simulink model "M2C_IM_CL_V1_NCADMM_Sim"  (R2023a)
settings: Solver=ode4  StartTime=0.0  StopTime=t_sim  FixedStep=tsim  RelTol=1e-3
model workspace (MAT data in the model file):
  global_can_baud_rate = '1000000'
  global_ip_addresses : object (value not decoded)
values from neighbouring files (symbols this model uses):
  A = [1 1 1 0 0 0 ... (first row only)    [M2C_init.m]    (also in MMCC_Sim_Script_BCD_activeset.m = -[1 0 0 1 0 0 1 0 0; 0 1 0 0 1 0 0 1 0; 0 0 1 0 0 1 0 0 1; -; MMCC_Sim_Script_BCD_activeset_LH.m = -[1 0 0 1 0 0 1 0 0; 0 1 0 0 1 0 0 1 0; 0 0 1 0 0 1 0 0 1; -)
  A11 = -(1/tau_sig)*eye(2)    [M2C_init.m]
  A21 = (Lm/tau_r)*eye(2)    [M2C_init.m]
  A_admm = zeros(2*Np, Np)    [M2C_init.m]
  A_cc = [1 0 ... (first row only)    [M2C_init.m]
  b_admm_1 = imax_admm*ones(2*Np,1)    [M2C_init.m]
  b_cc = Vmax_cc*ones(4,1)    [M2C_init.m]
  c_admm = -imax_admm*ones(Np,1)    [M2C_init.m]
  C_obs = [eye(2) zeros(2)]    [M2C_init.m]
  C_sm = 987e-6    (= 0.000987)    [M2C_init.m]
  G_cc = [1 1 ... (first row only)    [M2C_init.m]
  J_imag = [0 -1 ... (first row only)    [M2C_init.m]
  K_obsm = K_obs2'    [M2C_init.m]
  K_obsp = K_obs1'    [M2C_init.m]
  kr = Lm/Lr    (= 0.989061842659)    [M2C_init.m]
  L = 5e-3    (= 0.005)    [M2C_init.m]    (also in MMCC_Sim_Script_BCD_activeset.m = 0.02; MMCC_Sim_Script_BCD_activeset_LH.m = 0.02)
  Lsigmar = 2.6e-3    (= 0.0026)    [M2C_init.m]
  Lsigmas = 2.6e-3    (= 0.0026)    [M2C_init.m]
  N = [1/sqrt(3) 0;-1/(2*sqrt(3)) 1/2;-1/(2*sqrt(3)) -1/2;-1/sqrt(3) 0;1/(2*sqrt(3)) -1/2;1/(2*sqrt(3)) 1/2]    [M2C_init.m]    (also in MMCC_Sim_Script_BCD_activeset.m = null(A,'rational'); MMCC_Sim_Script_BCD_activeset_LH.m = [-0.4430   -0.4780    0.0994    0.0994)
  n = 4    [M2C_init.m]
  p = 2    [M2C_init.m]
  phirN = 1*Vb/ws_nom    [M2C_init.m]
  prmt_ADMM = [n, lambda_z, rho, lambda_e, C_sm, Np, imax_admm]    [M2C_init.m]
  prmt_bkpsi = [ts, Np, lambda_o, imax_admm]    [M2C_init.m]
  prmt_CCMPC = [ts, L, lambda_u, lambda_i, R, e]    [M2C_init.m]
  prmt_OBS = [ts, kr, sigma, Ls, tau_r]    [M2C_init.m]
  R = 0.2    [M2C_init.m]    (also in MMCC_Sim_Script_BCD_activeset.m = 0.001; MMCC_Sim_Script_BCD_activeset_LH.m = 0.001)
  Rr = 1.8    [M2C_init.m]
  Rs = 1.8    [M2C_init.m]
  Rsig = Rs + Rr*kr^2    (= 3.56083799149)    [M2C_init.m]
  SN = PN/FPn    (= 3703.7037037)    [M2C_init.m]
  T = [An ... (first row only)    [M2C_init.m]    (also in MMCC_Sim_Script_BCD_activeset.m = [1   0 ; -1/2  sqrt(3)/2; -1/2  -sqrt(3)/2]; MMCC_Sim_Script_BCD_activeset_LH.m = [1   0 ; -1/2  sqrt(3)/2; -1/2  -sqrt(3)/2])
  t_arranque = t_flux + 5/(dam*wn_flux) + 0.4    [M2C_init.m]
  t_flux = t_maq + 0.1    (= 0.3)    [M2C_init.m]
  t_load = t_arranque    [M2C_init.m]
  Tab0 = (1/3)*[2 -1 -1 ... (first row only)    [M2C_init.m]
  Tabc = [1 0; -.5 sqrt(3)/2; -.5 -sqrt(3)/2]    [M2C_init.m]
  tau_r = Lr/Rr    (= 0.132055555556)    [M2C_init.m]
  TN = PN/(nN*pi/30)    (= 19.7571653493)    [M2C_init.m]
  ts = 1/fs    (= 0.000166666666667)    [M2C_init.m]
  tsim = ts/40    (= 4.16666666667e-06)    [M2C_init.m]
  Vc0 = n*Vc_sm    (= 520)    [M2C_init.m]    (also in MMCC_Sim_Script_BCD_activeset.m = 18000; MMCC_Sim_Script_BCD_activeset_LH.m = 18000)
  Vc_sm = 130    [M2C_init.m]
  Vdc = n*Vc_sm    (= 520)    [M2C_init.m]
undefined symbols (not defined in the file or in its folder): Down, M2C_ADMM_Init_IM_V1, plecs, Up
libraries: spsIGBTDiodeLib x48, spsVoltageMeasurementLib x36, spsSeriesRLCBranchLib x30, spsCurrentMeasurementLib x10, eePwmGenerator x6, rtlab x3, dspstat3 x2, spsControlledVoltageSourceLib x2, spsDCVoltageSourceLib x2, opal_lib x1, dspfdesign x1, spsMeanLib x1
(part 3 of 6)

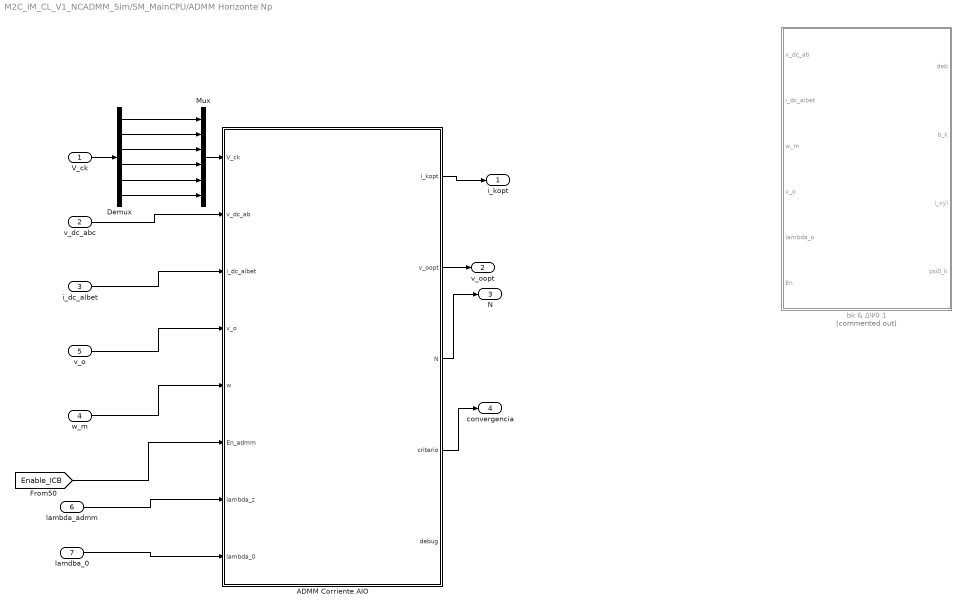
== system M2C_IM_CL_V1_NCADMM_Sim/SM_MainCPU/ADMM Horizonte Np ==
  V_ck : Inport
  v_dc_abc : Inport  Port=2
  i_dc_albet : Inport  Port=3
  w_m : Inport  Port=4
  v_o : Inport  Port=5
  lambda_admm : Inport  Port=6
  lamdba_0 : Inport  Port=7
  ADMM Corriente AIO : MATLAB Function  TreatAsAtomicUnit=on  SystemSampleTime=ts
  Demux : Demux  Outputs=6
  Mux : Mux  Inputs=6
  bk & ΔΨ0 1 : MATLAB Function  Commented=on  TreatAsAtomicUnit=on  SystemSampleTime=ts
  i_kopt : Outport
  v_oopt : Outport  Port=2
  N : Outport  Port=3
  convergencia : Outport  Port=4
  wires:
  V_ck/1 -> Demux/1
  Demux/1 -> Mux/1
  Demux/2 -> Mux/2
  Demux/3 -> Mux/3
  Demux/4 -> Mux/4
  Demux/5 -> Mux/5
  Demux/6 -> Mux/6
  v_o/1 -> ADMM Corriente AIO/4(v_o)
  i_dc_albet/1 -> ADMM Corriente AIO/3(i_dc_albet)
  v_dc_abc/1 -> ADMM Corriente AIO/2(v_dc_ab)
  ADMM Corriente AIO/1(i_kopt) -> i_kopt/1
  ADMM Corriente AIO/3(N) -> N/1
  ADMM Corriente AIO/4(criterio) -> convergencia/1
  [Enable_ICB] -> ADMM Corriente AIO/6(En_admm)
  w_m/1 -> ADMM Corriente AIO/5(w)
  Mux/1 -> ADMM Corriente AIO/1(V_ck)
  lambda_admm/1 -> ADMM Corriente AIO/7(lambda_z)
  lamdba_0/1 -> ADMM Corriente AIO/8(lambda_0)
  ADMM Corriente AIO/2(v_oopt) -> v_oopt/1

== system M2C_IM_CL_V1_NCADMM_Sim/SM_MainCPU/Corrientes ==
  1 : Inport
  2 : Inport  Port=2
  3 : Inport  Port=3
  4 : Inport  Port=4
  " 1 " : DataTypeConversion
  " 2 " : DataTypeConversion
  " 3 " : DataTypeConversion
  " 4 " : DataTypeConversion
  " InputMux " : Mux
  " S-Function " : S-Function  FunctionName=plecs  SFunctionDeploymentMode=off  EnableBusSupport=off
  wires:
  " InputMux "/1 -> " S-Function "/1
  1/1 -> " 1 "/1
  " 1 "/1 -> " InputMux "/1
  2/1 -> " 2 "/1
  " 2 "/1 -> " InputMux "/2
  3/1 -> " 3 "/1
  " 3 "/1 -> " InputMux "/3
  4/1 -> " 4 "/1
  " 4 "/1 -> " InputMux "/4

== system M2C_IM_CL_V1_NCADMM_Sim/SM_MainCPU/Entrada ==
  1 : Inport
  2 : Inport  Port=2
  " 1 " : DataTypeConversion
  " 2 " : DataTypeConversion
  " InputMux " : Mux  Inputs=2
  " S-Function " : S-Function  FunctionName=plecs  SFunctionDeploymentMode=off  EnableBusSupport=off
  wires:
  " InputMux "/1 -> " S-Function "/1
  1/1 -> " 1 "/1
  " 1 "/1 -> " InputMux "/1
  2/1 -> " 2 "/1
  " 2 "/1 -> " InputMux "/2

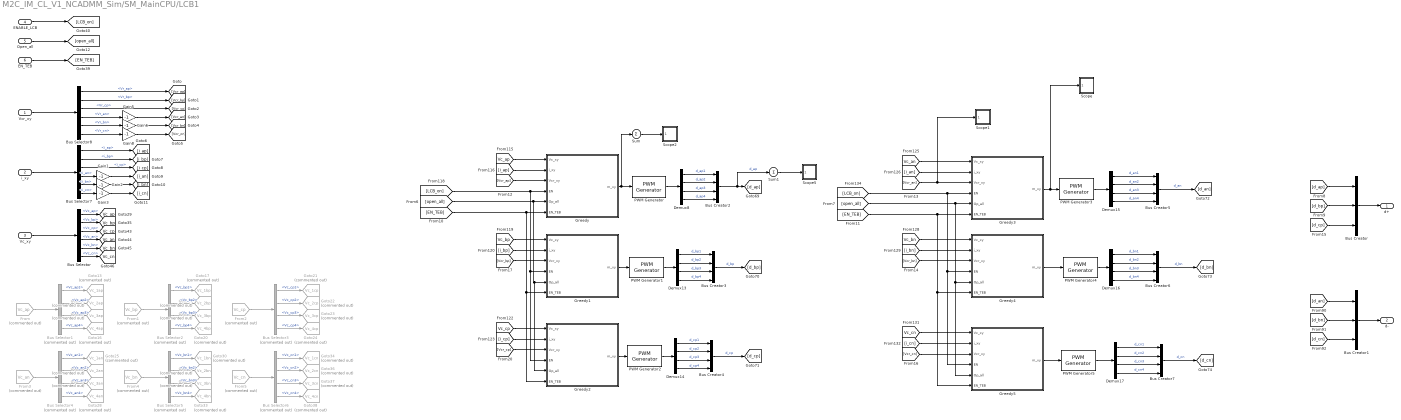
== system M2C_IM_CL_V1_NCADMM_Sim/SM_MainCPU/LCB1 ==
  Vcr_xy : Inport
  i_xy : Inport  Port=2
  Vc_xy : Inport  Port=3
  ENABLE_LCB : Inport  Port=4
  Open_all : Inport  Port=5
  EN_TEB : Inport  Port=6
  Bus Creator : BusCreator  Inputs=3
  Bus Creator1 : BusCreator  Inputs=3
  Bus Creator{2..7} (6 alike) : BusCreator  Inputs=4
  Bus Selector : BusSelector  OutputSignals=Vc_ap,Vc_bp,Vc_cp,Vc_an,Vc_bn,Vc_cn
  Bus Selector1 : BusSelector  Commented=on  OutputSignals=Vc_ap1,Vc_ap2,Vc_ap3,Vc_ap4
  Bus Selector2 : BusSelector  Commented=on  OutputSignals=Vc_bp1,Vc_bp2,Vc_bp3,Vc_bp4
  Bus Selector3 : BusSelector  Commented=on  OutputSignals=Vc_cp1,Vc_cp2,Vc_cp3,Vc_cp4
  Bus Selector4 : BusSelector  Commented=on  OutputSignals=Vc_an1,Vc_an2,Vc_an3,Vc_an4
  Bus Selector5 : BusSelector  Commented=on  OutputSignals=Vc_bn1,Vc_bn2,Vc_bn3,Vc_bn4
  Bus Selector6 : BusSelector  Commented=on  OutputSignals=Vc_cn1,Vc_cn2,Vc_cn3,Vc_cn4
  Bus Selector7 : BusSelector  OutputSignals=i_ap,i_bp,i_cp,i_an,i_bn,i_cn
  Bus Selector8 : BusSelector  OutputSignals=Vr_ap,Vr_bp,Vr_cp,Vr_an,Vr_bn,Vr_cn
  Demux{8,13..17} (6 alike) : Demux
  From : From  Commented=on  GotoTag=Vc_ap  TagVisibility=global
  From1 : From  Commented=on  GotoTag=Vc_bp  TagVisibility=global
  From2 : From  Commented=on  GotoTag=Vc_cp  TagVisibility=global
  From3 : From  Commented=on  GotoTag=Vc_an  TagVisibility=global
  From4 : From  Commented=on  GotoTag=Vc_bn  TagVisibility=global
  From5 : From  Commented=on  GotoTag=Vc_cn  TagVisibility=global
  Gain{1..3,5..6,8} (6 alike) : Gain  Gain=-1
  Goto13 : Goto  Commented=on  GotoTag=Vc_1ap  TagVisibility=global
  Goto14 : Goto  Commented=on  GotoTag=Vc_2ap  TagVisibility=global
  Goto15 : Goto  Commented=on  GotoTag=Vc_3ap  TagVisibility=global
  Goto16 : Goto  Commented=on  GotoTag=Vc_4ap  TagVisibility=global
  Goto17 : Goto  Commented=on  GotoTag=Vc_1bp  TagVisibility=global
  Goto18 : Goto  Commented=on  GotoTag=Vc_2bp  TagVisibility=global
  Goto19 : Goto  Commented=on  GotoTag=Vc_3bp  TagVisibility=global
  Goto20 : Goto  Commented=on  GotoTag=Vc_4bp  TagVisibility=global
  Goto21 : Goto  Commented=on  GotoTag=Vc_1cp  TagVisibility=global
  Goto22 : Goto  Commented=on  GotoTag=Vc_2cp  TagVisibility=global
  Goto23 : Goto  Commented=on  GotoTag=Vc_3cp  TagVisibility=global
  Goto24 : Goto  Commented=on  GotoTag=Vc_4cp  TagVisibility=global
  Goto25 : Goto  Commented=on  GotoTag=Vc_1an  TagVisibility=global
  Goto26 : Goto  Commented=on  GotoTag=Vc_2an  TagVisibility=global
  Goto27 : Goto  Commented=on  GotoTag=Vc_3an  TagVisibility=global
  Goto28 : Goto  Commented=on  GotoTag=Vc_4an  TagVisibility=global
  Goto30 : Goto  Commented=on  GotoTag=Vc_1bn  TagVisibility=global
  Goto31 : Goto  Commented=on  GotoTag=Vc_2bn  TagVisibility=global
  Goto32 : Goto  Commented=on  GotoTag=Vc_3bn  TagVisibility=global
  Goto33 : Goto  Commented=on  GotoTag=Vc_4bn  TagVisibility=global
  Goto34 : Goto  Commented=on  GotoTag=Vc_1cn  TagVisibility=global
  Goto36 : Goto  Commented=on  GotoTag=Vc_2cn  TagVisibility=global
  Goto37 : Goto  Commented=on  GotoTag=Vc_3cn  TagVisibility=global
  Goto38 : Goto  Commented=on  GotoTag=Vc_4cn  TagVisibility=global
  Greedy : MATLAB Function  TreatAsAtomicUnit=on
  Greedy1 : MATLAB Function  TreatAsAtomicUnit=on
  Greedy2 : MATLAB Function  TreatAsAtomicUnit=on
  Greedy3 : MATLAB Function  TreatAsAtomicUnit=on
  Greedy4 : MATLAB Function  TreatAsAtomicUnit=on
  Greedy5 : MATLAB Function  TreatAsAtomicUnit=on
  PWM Generator{,1..5} (6 alike) : eePwmGenerator/PWM Generator  CarrCount=Up-Down  Tper=ts*0.5  Tdelay=0  Ts=tsim
  Scope : Subsystem  LoadFcn=plecs('sl', 300);  InitFcn=plecs('sl', 314);  StartFcn=plecs('sl', 308);  StopFcn=plecs('sl', 309);  mask{Settings=<binary blob, 1052 chars, not shown>}
      mask init:
      | plecs('sl', 315);
      settings: CopyFcn=plecs('sl', 303);  DeleteFcn=plecs('sl', 305);  UndoDeleteFcn=plecs('sl', 306);  PreSaveFcn=plecs('sl', 311);  NameChangeFcn=plecs('sl', 310);  DestroyFcn=plecs('sl', 307);  OpenFcn=plecs('sl', 302);  ErrorFcn=plerrorfcn
      mask Display: plot([0.1 0.9 0.9 0.1 0.1], [0.9 0.9 0.5 0.5 0.9])
  Scope1 : Subsystem  LoadFcn=plecs('sl', 300);  InitFcn=plecs('sl', 314);  StartFcn=plecs('sl', 308);  StopFcn=plecs('sl', 309);  mask{Settings=<binary blob, 1052 chars, not shown>}
      mask init:
      | plecs('sl', 315);
      settings: CopyFcn=plecs('sl', 303);  DeleteFcn=plecs('sl', 305);  UndoDeleteFcn=plecs('sl', 306);  PreSaveFcn=plecs('sl', 311);  NameChangeFcn=plecs('sl', 310);  DestroyFcn=plecs('sl', 307);  OpenFcn=plecs('sl', 302);  ErrorFcn=plerrorfcn
      mask Display: plot([0.1 0.9 0.9 0.1 0.1], [0.9 0.9 0.5 0.5 0.9])
  Scope2 : Subsystem  LoadFcn=plecs('sl', 300);  InitFcn=plecs('sl', 314);  StartFcn=plecs('sl', 308);  StopFcn=plecs('sl', 309);  mask{Settings=<binary blob, 1020 chars, not shown>}
      mask init:
      | plecs('sl', 315);
      settings: CopyFcn=plecs('sl', 303);  DeleteFcn=plecs('sl', 305);  UndoDeleteFcn=plecs('sl', 306);  PreSaveFcn=plecs('sl', 311);  NameChangeFcn=plecs('sl', 310);  DestroyFcn=plecs('sl', 307);  OpenFcn=plecs('sl', 302);  ErrorFcn=plerrorfcn
      mask Display: plot([0.1 0.9 0.9 0.1 0.1], [0.9 0.9 0.5 0.5 0.9])
  Scope5 : Subsystem  LoadFcn=plecs('sl', 300);  InitFcn=plecs('sl', 314);  StartFcn=plecs('sl', 308);  StopFcn=plecs('sl', 309);  mask{Settings=<binary blob, 1020 chars, not shown>}
      mask init:
      | plecs('sl', 315);
      settings: CopyFcn=plecs('sl', 303);  DeleteFcn=plecs('sl', 305);  UndoDeleteFcn=plecs('sl', 306);  PreSaveFcn=plecs('sl', 311);  NameChangeFcn=plecs('sl', 310);  DestroyFcn=plecs('sl', 307);  OpenFcn=plecs('sl', 302);  ErrorFcn=plerrorfcn
      mask Display: plot([0.1 0.9 0.9 0.1 0.1], [0.9 0.9 0.5 0.5 0.9])
  Sum : Sum  Inputs=+
  Sum1 : Sum  Inputs=+
  d+ : Outport
  d- : Outport  Port=2
  tag scope: Vc_an=global, Vc_ap=global, Vc_bn=global, Vc_bp=global, Vc_cn=global, Vc_cp=global
  wires:
  Bus Creator1/1 -> d-/1
  Bus Selector8/5 -> Gain6/1  "<Vr_bn>"
  Bus Selector8/6 -> Gain8/1  "<Vr_cn>"
  Bus Selector8/4 -> Gain5/1  "<Vr_an>"
  Bus Creator/1 -> d+/1
  Gain3/1 -> [i_cn]
  Gain2/1 -> [i_bn]
  Gain1/1 -> [i_an]
  Bus Selector7/3 -> [i_cp]  "<i_cp>"
  Bus Selector7/2 -> [i_bp]  "<i_bp>"
  Bus Selector7/1 -> [i_ap]  "<i_ap>"
  Bus Selector7/4 -> Gain1/1  "<i_an>"
  Bus Selector7/6 -> Gain3/1  "<i_cn>"
  Bus Selector7/5 -> Gain2/1  "<i_bn>"
  Bus Selector/3 -> [Vc_cp]  "<Vc_cp>"
  Bus Selector/2 -> [Vc_bp]  "<Vc_bp>"
  Bus Selector/6 -> [Vc_cn]  "<Vc_cn>"
  Bus Selector/4 -> [Vc_an]  "<Vc_an>"
  Bus Selector/5 -> [Vc_bn]  "<Vc_bn>"
  Bus Selector/1 -> [Vc_ap]  "<Vc_ap>"
  Bus Selector1/1 -> Goto13/1  "<Vc_ap1>"
  Bus Selector1/2 -> Goto14/1  "<Vc_ap2>"
  Bus Selector1/3 -> Goto15/1  "<Vc_ap3>"
  Bus Selector1/4 -> Goto16/1  "<Vc_ap4>"
  Bus Selector2/4 -> Goto20/1  "<Vc_bp4>"
  Bus Selector2/2 -> Goto18/1  "<Vc_bp2>"
  Bus Selector2/1 -> Goto17/1  "<Vc_bp1>"
  Bus Selector2/3 -> Goto19/1  "<Vc_bp3>"
  Bus Selector3/4 -> Goto24/1  "<Vc_cp4>"
  Bus Selector3/2 -> Goto22/1  "<Vc_cp2>"
  Bus Selector3/1 -> Goto21/1  "<Vc_cp1>"
  Bus Selector3/3 -> Goto23/1  "<Vc_cp3>"
  Bus Selector4/4 -> Goto28/1  "<Vc_an4>"
  Bus Selector4/2 -> Goto26/1  "<Vc_an2>"
  Bus Selector4/1 -> Goto25/1  "<Vc_an1>"
  Bus Selector4/3 -> Goto27/1  "<Vc_an3>"
  Bus Selector5/4 -> Goto33/1  "<Vc_bn4>"
  Bus Selector5/2 -> Goto31/1  "<Vc_bn2>"
  Bus Selector5/1 -> Goto30/1  "<Vc_bn1>"
  Bus Selector5/3 -> Goto32/1  "<Vc_bn3>"
  Bus Selector6/4 -> Goto38/1  "<Vc_cn4>"
  Bus Selector6/2 -> Goto36/1  "<Vc_cn2>"
  Bus Selector6/1 -> Goto34/1  "<Vc_cn1>"
  Bus Selector6/3 -> Goto37/1  "<Vc_cn3>"
  [d_ap] -> Bus Creator/1
  [d_bp] -> Bus Creator/2
  [d_cp] -> Bus Creator/3
  [d_an] -> Bus Creator1/1
  [d_bn] -> Bus Creator1/2
  [d_cn] -> Bus Creator1/3
  [Vc_ap] -> Greedy/1(Vc_xy)
  [i_ap] -> Greedy/2(i_xy)
  Bus Selector8/2 -> [Vcr_bp]  "<Vr_bp>"
  Bus Selector8/3 -> [Vcr_cp]  "<Vr_cp>"
  Gain5/1 -> [Vcr_an]
  Gain6/1 -> [Vcr_bn]
  Gain8/1 -> [Vcr_cn]
  Bus Selector8/1 -> [Vcr_ap]  "<Vr_ap>"
  [Vcr_ap] -> Greedy/3(Vcr_xy)
  Vcr_xy/1 -> Bus Selector8/1
  Demux15/1 -> Bus Creator5/1  "d_an1"
  Demux15/2 -> Bus Creator5/2  "d_an2"
  Demux15/3 -> Bus Creator5/3  "d_an3"
  Demux15/4 -> Bus Creator5/4  "d_an4"
  Bus Creator5/1 -> [d_an]  "d_an"
  Demux8/3 -> Bus Creator2/3  "d_ap3"
  Demux8/1 -> Bus Creator2/1  "d_ap1"
  Demux8/2 -> Bus Creator2/2  "d_ap2"
  Demux8/4 -> Bus Creator2/4  "d_ap4"
  Demux13/4 -> Bus Creator3/4  "d_bp4"
  Demux13/2 -> Bus Creator3/2  "d_bp2"
  Demux13/1 -> Bus Creator3/1  "d_bp1"
  Demux13/3 -> Bus Creator3/3  "d_bp3"
  Demux14/3 -> Bus Creator4/3  "d_cp3"
  Demux14/1 -> Bus Creator4/1  "d_cp1"
  Demux14/2 -> Bus Creator4/2  "d_cp2"
  Demux14/4 -> Bus Creator4/4  "d_cp4"
  Bus Creator4/1 -> [d_cp]  "d_cp"
  Bus Creator3/1 -> [d_bp]  "d_bp"
  Bus Creator2/1 -> Sum1/1, [d_ap]  "d_ap"
  Bus Creator6/1 -> [d_bn]  "d_bn"
  Demux16/4 -> Bus Creator6/4  "d_bn4"
  Demux16/3 -> Bus Creator6/3  "d_bn3"
  Demux16/2 -> Bus Creator6/2  "d_bn2"
  Demux16/1 -> Bus Creator6/1  "d_bn1"
  Demux17/1 -> Bus Creator7/1  "d_cn1"
  Demux17/2 -> Bus Creator7/2  "d_cn2"
  Demux17/3 -> Bus Creator7/3  "d_cn3"
  Demux17/4 -> Bus Creator7/4  "d_cn4"
  Bus Creator7/1 -> [d_cn]  "d_cn"
  Vc_xy/1 -> Bus Selector/1
  From/1 -> Bus Selector1/1
  From1/1 -> Bus Selector2/1
  From2/1 -> Bus Selector3/1
  From3/1 -> Bus Selector4/1
  From4/1 -> Bus Selector5/1
  From5/1 -> Bus Selector6/1
  i_xy/1 -> Bus Selector7/1
  ENABLE_LCB/1 -> [LCB_on]
  Greedy/1(m_xy) -> Sum/1, PWM Generator/1
  Open_all/1 -> [open_all]
  Greedy1/1(m_xy) -> PWM Generator1/1
  Greedy2/1(m_xy) -> PWM Generator2/1
  [LCB_on] -> Greedy/4(EN), Greedy2/4(EN), Greedy1/4(EN)
  [open_all] -> Greedy2/5(Op_all), Greedy1/5(Op_all), Greedy/5(Op_all)
  EN_TEB/1 -> [EN_TEB]
  [EN_TEB] -> Greedy2/6(EN_TEB), Greedy1/6(EN_TEB), Greedy/6(EN_TEB)
  [Vc_bp] -> Greedy1/1(Vc_xy)
  [i_bp] -> Greedy1/2(i_xy)
  [Vcr_bp] -> Greedy1/3(Vcr_xy)
  [Vc_cp] -> Greedy2/1(Vc_xy)
  [i_cp] -> Greedy2/2(i_xy)
  [Vcr_cp] -> Greedy2/3(Vcr_xy)
  Greedy3/1(m_xy) -> Scope/1(1), PWM Generator3/1
  [Vc_an] -> Greedy3/1(Vc_xy)
  [i_an] -> Greedy3/2(i_xy)
  [Vcr_an] -> Scope1/1(1), Greedy3/3(Vcr_xy)
  [EN_TEB] -> Greedy3/6(EN_TEB), Greedy5/6(EN_TEB), Greedy4/6(EN_TEB)
  [LCB_on] -> Greedy3/4(EN), Greedy5/4(EN), Greedy4/4(EN)
  [open_all] -> Greedy3/5(Op_all), Greedy5/5(Op_all), Greedy4/5(Op_all)
  Greedy4/1(m_xy) -> PWM Generator4/1
  [Vc_bn] -> Greedy4/1(Vc_xy)
  [i_bn] -> Greedy4/2(i_xy)
  [Vcr_bn] -> Greedy4/3(Vcr_xy)
  Greedy5/1(m_xy) -> PWM Generator5/1
  [Vc_cn] -> Greedy5/1(Vc_xy)
  [i_cn] -> Greedy5/2(i_xy)
  [Vcr_cn] -> Greedy5/3(Vcr_xy)
  PWM Generator/1 -> Demux8/1
  PWM Generator1/1 -> Demux13/1
  PWM Generator2/1 -> Demux14/1
  PWM Generator3/1 -> Demux15/1
  PWM Generator4/1 -> Demux16/1
  PWM Generator5/1 -> Demux17/1
  Sum/1 -> Scope2/1(1)
  Sum1/1 -> Scope5/1(1)

== system M2C_IM_CL_V1_NCADMM_Sim/SM_MainCPU/Salida ==
  1 : Inport
  2 : Inport  Port=2
  3 : Inport  Port=3
  4 : Inport  Port=4
  5 : Inport  Port=5
  " 1 " : DataTypeConversion
  " 2 " : DataTypeConversion
  " 3 " : DataTypeConversion
  " 4 " : DataTypeConversion
  " 5 " : DataTypeConversion
  " InputMux " : Mux  Inputs=5
  " S-Function " : S-Function  FunctionName=plecs  SFunctionDeploymentMode=off  EnableBusSupport=off
  wires:
  " InputMux "/1 -> " S-Function "/1
  1/1 -> " 1 "/1
  " 1 "/1 -> " InputMux "/1
  2/1 -> " 2 "/1
  " 2 "/1 -> " InputMux "/2
  3/1 -> " 3 "/1
  " 3 "/1 -> " InputMux "/3
  4/1 -> " 4 "/1
  " 4 "/1 -> " InputMux "/4
  5/1 -> " 5 "/1
  " 5 "/1 -> " InputMux "/5

== system M2C_IM_CL_V1_NCADMM_Sim/SM_MainCPU/Scope ==
  1 : Inport
  " InputMux " : Subsystem
      mask Display: disp('Mux')
  " S-Function " : S-Function  FunctionName=plecs  SFunctionDeploymentMode=off  EnableBusSupport=off
  wires:
  1/1 -> " InputMux "/1(In1)
  " InputMux "/1(Out) -> " S-Function "/1

== system M2C_IM_CL_V1_NCADMM_Sim/SM_MainCPU/Scope1 ==
  1 : Inport
  " InputMux " : Subsystem
      mask Display: disp('Mux')
  " S-Function " : S-Function  FunctionName=plecs  SFunctionDeploymentMode=off  EnableBusSupport=off
  wires:
  1/1 -> " InputMux "/1(In1)
  " InputMux "/1(Out) -> " S-Function "/1

== system M2C_IM_CL_V1_NCADMM_Sim/SM_MainCPU/Scope10 ==
  1 : Inport
  " InputMux " : Subsystem
      mask Display: disp('Mux')
  " S-Function " : S-Function  FunctionName=plecs  SFunctionDeploymentMode=off  EnableBusSupport=off
  wires:
  1/1 -> " InputMux "/1(In1)
  " InputMux "/1(Out) -> " S-Function "/1

== system M2C_IM_CL_V1_NCADMM_Sim/SM_MainCPU/Scope11 ==
  1 : Inport
  " InputMux " : Subsystem
      mask Display: disp('Mux')
  " S-Function " : S-Function  FunctionName=plecs  SFunctionDeploymentMode=off  EnableBusSupport=off
  wires:
  1/1 -> " InputMux "/1(In1)
  " InputMux "/1(Out) -> " S-Function "/1

== system M2C_IM_CL_V1_NCADMM_Sim/SM_MainCPU/Scope12 ==
  1 : Inport
  " InputMux " : Subsystem
      mask Display: disp('Mux')
  " S-Function " : S-Function  FunctionName=plecs  SFunctionDeploymentMode=off  EnableBusSupport=off
  wires:
  1/1 -> " InputMux "/1(In1)
  " InputMux "/1(Out) -> " S-Function "/1

== system M2C_IM_CL_V1_NCADMM_Sim/SM_MainCPU/Scope13 ==
  1 : Inport
  " InputMux " : Subsystem
      mask Display: disp('Mux')
  " S-Function " : S-Function  FunctionName=plecs  SFunctionDeploymentMode=off  EnableBusSupport=off
  wires:
  1/1 -> " InputMux "/1(In1)
  " InputMux "/1(Out) -> " S-Function "/1

== system M2C_IM_CL_V1_NCADMM_Sim/SM_MainCPU/Scope14 ==
  1 : Inport
  " InputMux " : Subsystem
      mask Display: disp('Mux')
  " S-Function " : S-Function  FunctionName=plecs  SFunctionDeploymentMode=off  EnableBusSupport=off
  wires:
  1/1 -> " InputMux "/1(In1)
  " InputMux "/1(Out) -> " S-Function "/1

== system M2C_IM_CL_V1_NCADMM_Sim/SM_MainCPU/Scope15 ==
  1 : Inport
  " InputMux " : Subsystem
      mask Display: disp('Mux')
  " S-Function " : S-Function  FunctionName=plecs  SFunctionDeploymentMode=off  EnableBusSupport=off
  wires:
  1/1 -> " InputMux "/1(In1)
  " InputMux "/1(Out) -> " S-Function "/1

== system M2C_IM_CL_V1_NCADMM_Sim/SM_MainCPU/Scope16 ==
  1 : Inport
  " InputMux " : Subsystem
      mask Display: disp('Mux')
  " S-Function " : S-Function  FunctionName=plecs  SFunctionDeploymentMode=off  EnableBusSupport=off
  wires:
  1/1 -> " InputMux "/1(In1)
  " InputMux "/1(Out) -> " S-Function "/1

== system M2C_IM_CL_V1_NCADMM_Sim/SM_MainCPU/Scope17 ==
  1 : Inport
  " InputMux " : Subsystem
      mask Display: disp('Mux')
  " S-Function " : S-Function  FunctionName=plecs  SFunctionDeploymentMode=off  EnableBusSupport=off
  wires:
  1/1 -> " InputMux "/1(In1)
  " InputMux "/1(Out) -> " S-Function "/1

== system M2C_IM_CL_V1_NCADMM_Sim/SM_MainCPU/Scope18 ==
  1 : Inport
  " InputMux " : Subsystem
      mask Display: disp('Mux')
  " S-Function " : S-Function  FunctionName=plecs  SFunctionDeploymentMode=off  EnableBusSupport=off
  wires:
  1/1 -> " InputMux "/1(In1)
  " InputMux "/1(Out) -> " S-Function "/1

== system M2C_IM_CL_V1_NCADMM_Sim/SM_MainCPU/Scope19 ==
  1 : Inport
  " InputMux " : Subsystem
      mask Display: disp('Mux')
  " S-Function " : S-Function  FunctionName=plecs  SFunctionDeploymentMode=off  EnableBusSupport=off
  wires:
  1/1 -> " InputMux "/1(In1)
  " InputMux "/1(Out) -> " S-Function "/1

== system M2C_IM_CL_V1_NCADMM_Sim/SM_MainCPU/Scope2 ==
  1 : Inport
  " InputMux " : Subsystem
      mask Display: disp('Mux')
  " S-Function " : S-Function  FunctionName=plecs  SFunctionDeploymentMode=off  EnableBusSupport=off
  wires:
  1/1 -> " InputMux "/1(In1)
  " InputMux "/1(Out) -> " S-Function "/1

== system M2C_IM_CL_V1_NCADMM_Sim/SM_MainCPU/Scope20 ==
  1 : Inport
  " InputMux " : Subsystem
      mask Display: disp('Mux')
  " S-Function " : S-Function  FunctionName=plecs  SFunctionDeploymentMode=off  EnableBusSupport=off
  wires:
  1/1 -> " InputMux "/1(In1)
  " InputMux "/1(Out) -> " S-Function "/1

== system M2C_IM_CL_V1_NCADMM_Sim/SM_MainCPU/Scope21 ==
  1 : Inport
  " InputMux " : Subsystem
      mask Display: disp('Mux')
  " S-Function " : S-Function  FunctionName=plecs  SFunctionDeploymentMode=off  EnableBusSupport=off
  wires:
  1/1 -> " InputMux "/1(In1)
  " InputMux "/1(Out) -> " S-Function "/1

== system M2C_IM_CL_V1_NCADMM_Sim/SM_MainCPU/Scope22 ==
  1 : Inport
  " InputMux " : Subsystem
      mask Display: disp('Mux')
  " S-Function " : S-Function  FunctionName=plecs  SFunctionDeploymentMode=off  EnableBusSupport=off
  wires:
  1/1 -> " InputMux "/1(In1)
  " InputMux "/1(Out) -> " S-Function "/1

== system M2C_IM_CL_V1_NCADMM_Sim/SM_MainCPU/Scope23 ==
  1 : Inport
  2 : Inport  Port=2
  3 : Inport  Port=3
  4 : Inport  Port=4
  5 : Inport  Port=5
  6 : Inport  Port=6
  " 1 " : DataTypeConversion
  " 2 " : DataTypeConversion
  " 3 " : DataTypeConversion
  " 4 " : DataTypeConversion
  " 5 " : DataTypeConversion
  " 6 " : DataTypeConversion
  " InputMux " : Mux  Inputs=6
  " S-Function " : S-Function  FunctionName=plecs  SFunctionDeploymentMode=off  EnableBusSupport=off
  wires:
  " InputMux "/1 -> " S-Function "/1
  1/1 -> " 1 "/1
  " 1 "/1 -> " InputMux "/1
  2/1 -> " 2 "/1
  " 2 "/1 -> " InputMux "/2
  3/1 -> " 3 "/1
  " 3 "/1 -> " InputMux "/3
  4/1 -> " 4 "/1
  " 4 "/1 -> " InputMux "/4
  5/1 -> " 5 "/1
  " 5 "/1 -> " InputMux "/5
  6/1 -> " 6 "/1
  " 6 "/1 -> " InputMux "/6

== system M2C_IM_CL_V1_NCADMM_Sim/SM_MainCPU/Scope24 ==
  1 : Inport
  " InputMux " : Subsystem
      mask Display: disp('Mux')
  " S-Function " : S-Function  FunctionName=plecs  SFunctionDeploymentMode=off  EnableBusSupport=off
  wires:
  1/1 -> " InputMux "/1(In1)
  " InputMux "/1(Out) -> " S-Function "/1

== system M2C_IM_CL_V1_NCADMM_Sim/SM_MainCPU/Scope25 ==
  1 : Inport
  " InputMux " : Subsystem
      mask Display: disp('Mux')
  " S-Function " : S-Function  FunctionName=plecs  SFunctionDeploymentMode=off  EnableBusSupport=off
  wires:
  1/1 -> " InputMux "/1(In1)
  " InputMux "/1(Out) -> " S-Function "/1

== system M2C_IM_CL_V1_NCADMM_Sim/SM_MainCPU/Scope26 ==
  1 : Inport
  " InputMux " : Subsystem
      mask Display: disp('Mux')
  " S-Function " : S-Function  FunctionName=plecs  SFunctionDeploymentMode=off  EnableBusSupport=off
  wires:
  1/1 -> " InputMux "/1(In1)
  " InputMux "/1(Out) -> " S-Function "/1

== system M2C_IM_CL_V1_NCADMM_Sim/SM_MainCPU/Scope27 ==
  1 : Inport
  " InputMux " : Subsystem
      mask Display: disp('Mux')
  " S-Function " : S-Function  FunctionName=plecs  SFunctionDeploymentMode=off  EnableBusSupport=off
  wires:
  1/1 -> " InputMux "/1(In1)
  " InputMux "/1(Out) -> " S-Function "/1

== system M2C_IM_CL_V1_NCADMM_Sim/SM_MainCPU/Scope28 ==
  1 : Inport
  " InputMux " : Subsystem
      mask Display: disp('Mux')
  " S-Function " : S-Function  FunctionName=plecs  SFunctionDeploymentMode=off  EnableBusSupport=off
  wires:
  1/1 -> " InputMux "/1(In1)
  " InputMux "/1(Out) -> " S-Function "/1

== system M2C_IM_CL_V1_NCADMM_Sim/SM_MainCPU/Scope29 ==
  1 : Inport
  " InputMux " : Subsystem
      mask Display: disp('Mux')
  " S-Function " : S-Function  FunctionName=plecs  SFunctionDeploymentMode=off  EnableBusSupport=off
  wires:
  1/1 -> " InputMux "/1(In1)
  " InputMux "/1(Out) -> " S-Function "/1

== system M2C_IM_CL_V1_NCADMM_Sim/SM_MainCPU/Scope3 ==
  1 : Inport
  " InputMux " : Subsystem
      mask Display: disp('Mux')
  " S-Function " : S-Function  FunctionName=plecs  SFunctionDeploymentMode=off  EnableBusSupport=off
  wires:
  1/1 -> " InputMux "/1(In1)
  " InputMux "/1(Out) -> " S-Function "/1

== system M2C_IM_CL_V1_NCADMM_Sim/SM_MainCPU/Scope30 ==
  1 : Inport
  " InputMux " : Subsystem
      mask Display: disp('Mux')
  " S-Function " : S-Function  FunctionName=plecs  SFunctionDeploymentMode=off  EnableBusSupport=off
  wires:
  1/1 -> " InputMux "/1(In1)
  " InputMux "/1(Out) -> " S-Function "/1

== system M2C_IM_CL_V1_NCADMM_Sim/SM_MainCPU/Scope31 ==
  1 : Inport
  " InputMux " : Subsystem
      mask Display: disp('Mux')
  " S-Function " : S-Function  FunctionName=plecs  SFunctionDeploymentMode=off  EnableBusSupport=off
  wires:
  1/1 -> " InputMux "/1(In1)
  " InputMux "/1(Out) -> " S-Function "/1

== system M2C_IM_CL_V1_NCADMM_Sim/SM_MainCPU/Scope32 ==
  1 : Inport
  2 : Inport  Port=2
  3 : Inport  Port=3
  4 : Inport  Port=4
  5 : Inport  Port=5
  6 : Inport  Port=6
  " 1 " : DataTypeConversion
  " 2 " : DataTypeConversion
  " 3 " : DataTypeConversion
  " 4 " : DataTypeConversion
  " 5 " : DataTypeConversion
  " 6 " : DataTypeConversion
  " InputMux " : Mux  Inputs=6
  " S-Function " : S-Function  FunctionName=plecs  SFunctionDeploymentMode=off  EnableBusSupport=off
  wires:
  " InputMux "/1 -> " S-Function "/1
  1/1 -> " 1 "/1
  " 1 "/1 -> " InputMux "/1
  2/1 -> " 2 "/1
  " 2 "/1 -> " InputMux "/2
  3/1 -> " 3 "/1
  " 3 "/1 -> " InputMux "/3
  4/1 -> " 4 "/1
  " 4 "/1 -> " InputMux "/4
  5/1 -> " 5 "/1
  " 5 "/1 -> " InputMux "/5
  6/1 -> " 6 "/1
  " 6 "/1 -> " InputMux "/6

== system M2C_IM_CL_V1_NCADMM_Sim/SM_MainCPU/Scope33 ==
  1 : Inport
  " InputMux " : Subsystem
      mask Display: disp('Mux')
  " S-Function " : S-Function  FunctionName=plecs  SFunctionDeploymentMode=off  EnableBusSupport=off
  wires:
  1/1 -> " InputMux "/1(In1)
  " InputMux "/1(Out) -> " S-Function "/1

== system M2C_IM_CL_V1_NCADMM_Sim/SM_MainCPU/Scope34 ==
  1 : Inport
  " InputMux " : Subsystem
      mask Display: disp('Mux')
  " S-Function " : S-Function  FunctionName=plecs  SFunctionDeploymentMode=off  EnableBusSupport=off
  wires:
  1/1 -> " InputMux "/1(In1)
  " InputMux "/1(Out) -> " S-Function "/1

== system M2C_IM_CL_V1_NCADMM_Sim/SM_MainCPU/Scope35 ==
  1 : Inport
  " InputMux " : Subsystem
      mask Display: disp('Mux')
  " S-Function " : S-Function  FunctionName=plecs  SFunctionDeploymentMode=off  EnableBusSupport=off
  wires:
  1/1 -> " InputMux "/1(In1)
  " InputMux "/1(Out) -> " S-Function "/1

== system M2C_IM_CL_V1_NCADMM_Sim/SM_MainCPU/Scope36 ==
  1 : Inport
  " InputMux " : Subsystem
      mask Display: disp('Mux')
  " S-Function " : S-Function  FunctionName=plecs  SFunctionDeploymentMode=off  EnableBusSupport=off
  wires:
  1/1 -> " InputMux "/1(In1)
  " InputMux "/1(Out) -> " S-Function "/1

== system M2C_IM_CL_V1_NCADMM_Sim/SM_MainCPU/Scope37 ==
  1 : Inport
  " InputMux " : Subsystem
      mask Display: disp('Mux')
  " S-Function " : S-Function  FunctionName=plecs  SFunctionDeploymentMode=off  EnableBusSupport=off
  wires:
  1/1 -> " InputMux "/1(In1)
  " InputMux "/1(Out) -> " S-Function "/1

== system M2C_IM_CL_V1_NCADMM_Sim/SM_MainCPU/Scope38 ==
  1 : Inport
  " InputMux " : Subsystem
      mask Display: disp('Mux')
  " S-Function " : S-Function  FunctionName=plecs  SFunctionDeploymentMode=off  EnableBusSupport=off
  wires:
  1/1 -> " InputMux "/1(In1)
  " InputMux "/1(Out) -> " S-Function "/1

== system M2C_IM_CL_V1_NCADMM_Sim/SM_MainCPU/Scope39 ==
  1 : Inport
  " InputMux " : Subsystem
      mask Display: disp('Mux')
  " S-Function " : S-Function  FunctionName=plecs  SFunctionDeploymentMode=off  EnableBusSupport=off
  wires:
  1/1 -> " InputMux "/1(In1)
  " InputMux "/1(Out) -> " S-Function "/1

== system M2C_IM_CL_V1_NCADMM_Sim/SM_MainCPU/Scope4 ==
  1 : Inport
  " InputMux " : Subsystem
      mask Display: disp('Mux')
  " S-Function " : S-Function  FunctionName=plecs  SFunctionDeploymentMode=off  EnableBusSupport=off
  wires:
  1/1 -> " InputMux "/1(In1)
  " InputMux "/1(Out) -> " S-Function "/1

== system M2C_IM_CL_V1_NCADMM_Sim/SM_MainCPU/Scope40 ==
  1 : Inport
  " InputMux " : Subsystem
      mask Display: disp('Mux')
  " S-Function " : S-Function  FunctionName=plecs  SFunctionDeploymentMode=off  EnableBusSupport=off
  wires:
  1/1 -> " InputMux "/1(In1)
  " InputMux "/1(Out) -> " S-Function "/1

== system M2C_IM_CL_V1_NCADMM_Sim/SM_MainCPU/Scope41 ==
  1 : Inport
  " InputMux " : Subsystem
      mask Display: disp('Mux')
  " S-Function " : S-Function  FunctionName=plecs  SFunctionDeploymentMode=off  EnableBusSupport=off
  wires:
  1/1 -> " InputMux "/1(In1)
  " InputMux "/1(Out) -> " S-Function "/1

== system M2C_IM_CL_V1_NCADMM_Sim/SM_MainCPU/Scope42 ==
  1 : Inport
  " InputMux " : Subsystem
      mask Display: disp('Mux')
  " S-Function " : S-Function  FunctionName=plecs  SFunctionDeploymentMode=off  EnableBusSupport=off
  wires:
  1/1 -> " InputMux "/1(In1)
  " InputMux "/1(Out) -> " S-Function "/1

== system M2C_IM_CL_V1_NCADMM_Sim/SM_MainCPU/Scope5 ==
  1 : Inport
  " InputMux " : Subsystem
      mask Display: disp('Mux')
  " S-Function " : S-Function  FunctionName=plecs  SFunctionDeploymentMode=off  EnableBusSupport=off
  wires:
  1/1 -> " InputMux "/1(In1)
  " InputMux "/1(Out) -> " S-Function "/1

== system M2C_IM_CL_V1_NCADMM_Sim/SM_MainCPU/Scope6 ==
  1 : Inport
  " InputMux " : Subsystem
      mask Display: disp('Mux')
  " S-Function " : S-Function  FunctionName=plecs  SFunctionDeploymentMode=off  EnableBusSupport=off
  wires:
  1/1 -> " InputMux "/1(In1)
  " InputMux "/1(Out) -> " S-Function "/1

== system M2C_IM_CL_V1_NCADMM_Sim/SM_MainCPU/Scope7 ==
  1 : Inport
  " InputMux " : Subsystem
      mask Display: disp('Mux')
  " S-Function " : S-Function  FunctionName=plecs  SFunctionDeploymentMode=off  EnableBusSupport=off
  wires:
  1/1 -> " InputMux "/1(In1)
  " InputMux "/1(Out) -> " S-Function "/1

== system M2C_IM_CL_V1_NCADMM_Sim/SM_MainCPU/Scope8 ==
  1 : Inport
  " InputMux " : Subsystem
      mask Display: disp('Mux')
  " S-Function " : S-Function  FunctionName=plecs  SFunctionDeploymentMode=off  EnableBusSupport=off
  wires:
  1/1 -> " InputMux "/1(In1)
  " InputMux "/1(Out) -> " S-Function "/1

== system M2C_IM_CL_V1_NCADMM_Sim/SM_MainCPU/Scope9 ==
  1 : Inport
  " InputMux " : Subsystem
      mask Display: disp('Mux')
  " S-Function " : S-Function  FunctionName=plecs  SFunctionDeploymentMode=off  EnableBusSupport=off
  wires:
  1/1 -> " InputMux "/1(In1)
  " InputMux "/1(Out) -> " S-Function "/1
